simulink model "QuadrotorSimulink_nk"  (R2018b)
settings: Solver=ode45  StartTime=0.0  StopTime=options.T_train  FixedStep=0.001  RelTol=1e-6
undefined symbols (not defined in the file or in its folder): options, Quad
libraries: neural x67, simulink x1
(part 5 of 5)

== system QuadrotorSimulink_nk/NN/Layer 3/Delays 1 ==
  "p{3}" : Inport  PortDimensions=30
      mask Display: e = 0.06;c1 = [120 230 180]/255;c2 = ([120 230 180]+0)/(256+128);c3 = ([120 230 180]+128)/(256+128);patch([0 1 1 0],[0 0 1 1],c1);patch([0 1 1 1-e 1-e 0+e],[0 0 1 1-e 0+e 0+e],c2);patch([0 0 1 1-e 0+e 0+e],[0 1 1 1-e 1-e 0+e],c3);plot([0 1 1 0 0],[0 0 1 1 0]);
  mux : Mux  Inputs=1
      mask Display: e = 0.06;c1 = [120 150 230]/255;c2 = ([120 150 230]+0)/383;c3 = ([120 150 230]+128)/383;patch([0 1 1 0],[0 0 1 1],c1);patch([0 1 1 1-e 1-e 0+e],[0 0 1 1-e 0+e 0+e],c2);patch([0 0 1 1-e 0+e 0+e],[0 1 1 1-e 1-e 0+e],c3);plot([0 1 1 0 0],[0 0 1 1 0]);disp('Mux')
  "pd{3,2}" : Outport
      mask Display: e = 0.06;c1 = [120 230 180]/255;c2 = ([120 230 180]+0)/(256+128);c3 = ([120 230 180]+128)/(256+128);patch([0 1 1 0],[0 0 1 1],c1);patch([0 1 1 1-e 1-e 0+e],[0 0 1 1-e 0+e 0+e],c2);patch([0 0 1 1-e 0+e 0+e],[0 1 1 1-e 1-e 0+e],c3);plot([0 1 1 0 0],[0 0 1 1 0]);
  wires:
  "p{3}"/1 -> mux/1
  mux/1 -> "pd{3,2}"/1

== system QuadrotorSimulink_nk/NN/Layer 3/LW{3,2} ==
  "ad{3,2}" : Inport  PortDimensions=30
      mask Display: e = 0.06;c1 = [120 230 180]/255;c2 = ([120 230 180]+0)/(256+128);c3 = ([120 230 180]+128)/(256+128);patch([0 1 1 0],[0 0 1 1],c1);patch([0 1 1 1-e 1-e 0+e],[0 0 1 1-e 0+e 0+e],c2);patch([0 0 1 1-e 0+e 0+e],[0 1 1 1-e 1-e 0+e],c3);plot([0 1 1 0 0],[0 0 1 1 0]);
  "IW{3,2}(1,:)'" : Constant  Value=[0.16399643208309999664606948499567806720733642578125;-0.03221139281619082861407576956480625085532665252685546875;0.71844753313801901217772183372289873659610748291015625;0.78263798788498573077987430224311538040637969970703125;-0.71299915258685697683205262364936061203479766845703125;0.304555836790654732570970963934087194502353668212890625;-0.383527143030407413615279210716835223138332366943359375;0.1762666859109161821006495074470876716077327728271484375;0.499085706940436912848468864467577077448368072509765625;-0.62911144187184919740474242644268088042736053466796875;-0.027555467051344657847256058857965399511158466339111328125;0.28339713308875980057877086437656544148921966552734375;-0.2546190120415927626851271270425058901309967041015625;-0.5992809375793164416990066456492058932781219482421875;-0.421787635076959210866931471173302270472049713134765625;-0.73932488741903867879301515131373889744281768798828125;0.61346821217145441895723934067063964903354644775390625;-0.210516608721366516032702520533348433673381805419921875;-0.278003142357851673605040332404314540326595306396484375;0.777757525061978594038691880996339023113250732421875;0.56946269213540945397511450210004113614559173583984375;-0.1570059417677545365865654503068071790039539337158203125;-0.61539302144485219514535856433212757110595703125;0.1669241397766821066728226696795900352299213409423828125;-0.6124955919569934348345441321725957095623016357421875;0.1519280649083070422467045546000008471310138702392578125;-0.30435192005138933524222011328674852848052978515625;-0.72754654168113963574882063767290674149990081787109375;-0.69182864592810722204063722529099322855472564697265625;0.5879909736161599287385115530923940241336822509765625]
      mask Display: e = 0.06;c1 = [120 150 230]/255;c2 = ([120 150 230]+0)/383;c3 = ([120 150 230]+128)/383;patch([0 1 1 0],[0 0 1 1],c1);patch([0 1 1 1-e 1-e 0+e],[0 0 1 1-e 0+e 0+e],c2);patch([0 0 1 1-e 0+e 0+e],[0 1 1 1-e 1-e 0+e],c3);plot([0 1 1 0 0],[0 0 1 1 0]);disp('weights');
  "IW{3,2}(2,:)'" : Constant  Value=[0.60739896667457438095283350776298902928829193115234375;-0.603855457245570104163334690383635461330413818359375;0.1358443006612404524435788744085584767162799835205078125;-0.470038992576660430433577175790560431778430938720703125;0.50764457213076574770838078620727173984050750732421875;0.86747025011116118964338284058612771332263946533203125;-0.33441895684965883273065401226631365716457366943359375;0.238797709545060354852097361799678765237331390380859375;0.7522717149965674199307841263362206518650054931640625;0.152315237562284655492561569190002046525478363037109375;-0.64370596007031577467927263569436036050319671630859375;0.92396492774599447983518984983675181865692138671875;-0.2071339586370490593036919335645507089793682098388671875;-0.57321106980673375286272630546591244637966156005859375;0.312537598350990541984373294326360337436199188232421875;-0.08032311515206909391384471064156969077885150909423828125;0.93797293243875168311518564223661087453365325927734375;0.435963668711713714376543293838039971888065338134765625;-0.13105458983652573667910701260552741587162017822265625;-0.579243832058234264792417889111675322055816650390625;-0.97070483373580762620491668712929822504520416259765625;-0.098264154511598977848052527406252920627593994140625;0.90515674889206121367379864750546403229236602783203125;-0.4846317022686978948087244134512729942798614501953125;-0.092773620885304330929699290209100581705570220947265625;-0.71883248778889929919699852689518593251705169677734375;-0.33906801948969544913126128449221141636371612548828125;-0.5195429247991736332323853275738656520843505859375;0.96348653983777821085965342717827297747135162353515625;-0.69159499648207656274934151952038519084453582763671875]
      mask Display: e = 0.06;c1 = [120 150 230]/255;c2 = ([120 150 230]+0)/383;c3 = ([120 150 230]+128)/383;patch([0 1 1 0],[0 0 1 1],c1);patch([0 1 1 1-e 1-e 0+e],[0 0 1 1-e 0+e 0+e],c2);patch([0 0 1 1-e 0+e 0+e],[0 1 1 1-e 1-e 0+e],c3);plot([0 1 1 0 0],[0 0 1 1 0]);disp('weights');
  Mux : Mux  Inputs=2
      mask Display: e = 0.06;c1 = [120 150 230]/255;c2 = ([120 150 230]+0)/383;c3 = ([120 150 230]+128)/383;patch([0 1 1 0],[0 0 1 1],c1);patch([0 1 1 1-e 1-e 0+e],[0 0 1 1-e 0+e 0+e],c2);patch([0 0 1 1-e 0+e 0+e],[0 1 1 1-e 1-e 0+e],c3);plot([0 1 1 0 0],[0 0 1 1 0]);disp('Mux');
  dotprod1 : neural/Weight Functions/dotprod
  dotprod2 : neural/Weight Functions/dotprod
  "lz{3,2}" : Outport
      mask Display: e = 0.06;c1 = [120 230 180]/255;c2 = ([120 230 180]+0)/(256+128);c3 = ([120 230 180]+128)/(256+128);patch([0 1 1 0],[0 0 1 1],c1);patch([0 1 1 1-e 1-e 0+e],[0 0 1 1-e 0+e 0+e],c2);patch([0 0 1 1-e 0+e 0+e],[0 1 1 1-e 1-e 0+e],c3);plot([0 1 1 0 0],[0 0 1 1 0]);
  wires:
  "IW{3,2}(1,:)'"/1 -> dotprod1/1
  "ad{3,2}"/1 -> dotprod1/2, dotprod2/2
  dotprod1/1 -> Mux/1
  "IW{3,2}(2,:)'"/1 -> dotprod2/1
  dotprod2/1 -> Mux/2
  Mux/1 -> "lz{3,2}"/1
